simulink model "Template"  (R2018a)
settings: Solver=FixedStepDiscrete  StartTime=0.0  StopTime=0.001  RelTol=1e-3
values from neighbouring files (symbols this model uses):
  T = 1/Fs    (= 5e-05)    [SimVar.m]
undefined symbols (not defined in the file or in its folder): fdesignblkfcn, gcbh, get
libraries: dspsrcs4 x1, dspxfrm3 x1, dspobslib x1
settings Model: Creator=Daniel  LastModifiedBy=Daniel
settings SolverCC: AutoInsertRateTranBlk=on
settings DataIOCC: LimitDataPoints=on  SaveOutput=off  SignalLogging=off  SaveTime=off
settings OptimizationCC: LifeSpan=inf  SimCompilerOptimization=on
settings DebuggingCC: AlgebraicLoopMsg=error  SingleTaskRateTransMsg=error  AllowSymbolicDim=off  SFUnexpectedBacktrackingDiag=warning  SFNoUnconditionalDefaultTransitionDiag=warning  SFExecutionAtInitializationDiag=none
settings CodeAppCC: StateflowObjectComments=on
settings GRTTargetCC: TargetLangStandard=C89/C90 (ANSI)  GeneratePreprocessorConditionals=Disable all
settings ConfigComp: CovMetricSettings=dw  CovHtmlReporting=on  CovSaveCumulativeToWorkspaceVar=on  CovSaveSingleToWorkspaceVar=on  CovExternalEMLEnable=off  CovSFcnEnable=off

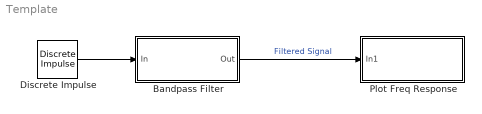
== system Template ==
  Bandpass Filter : Subsystem  DialogController=fdesignblkfcn  InitFcn=fdesignblkfcn(gcbh, {'InitFcn'});  mask(Bandpass Filter){}
      mask help: Design a bandpass filter
      settings: CopyFcn=fdesignblkfcn(gcbh, {'CopyFcn'});
      mask Help: helpview(mapfilelocation('dsp'), 'dspbandpassfilter');
      mask Display: disp('Bandpass');
  Discrete Impulse : dspsrcs4/Discrete  Impulse  Delay=0  SampleTime=T  FrameSample=128  OutputFrames=off  dataType=double  isSigned=on  wordLen=16  udDataType=sfix(16)  fracBitsMode=Best precision  numFracBits=15  OutDataTypeStr=double  LastOutDataTypeStr=double
  Plot Freq Response : Subsystem
  wires:
  Discrete Impulse/1 -> Bandpass Filter/1(In)
  Bandpass Filter/1(Out) -> Plot Freq Response/1(In1)  "Filtered Signal"

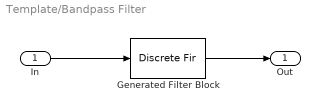
== system Template/Bandpass Filter ==
  In : Inport
  Generated Filter Block : DiscreteFir  Tag=BlockMethodSubSystem  Coefficients=[-0.0143829707087432795 -0.0290029983982484744 0.00784048811812495389 0.0308165601876585482 0.00100231088912336496 0.0087190389177637332 0.0151927377592376723 -0.00168387668084986558 0.0111183190197781962 0.00421002856557019852 0.000673765264122200562 0.00910146591908392137 -0.00227014796668174043 0.00546863785810260041 0.00231714434328688865 -0.00136078413445314315 0.00603880317721489351 -0.00343031068051817024 0.00347055870875673288 0.000464183487342060218 -0.00250956115928813303 0.00433762157606339387 -0.00498706380103555377 0.00246050102483365242 -0.00143811368573451407 -0.00366854398739842411 0.00299692463358692748 -0.00698080238922849181 0.0016607418180266374 -0.00363600133190109583 -0.00501339083555271074 0.00160027598954386673 -0.0094321788660009908 0.000886295582407861356 -0.00628897746187223605 -0.0065194850954027302 5.11766740212844773e-05 -0.0123554859169431042 0.000164116634503716995 -0.00940416859225592754 -0.00812346347120297338 -0.00168137988191204078 -0.015663036767903888 -0.000418207004173260346 -0.0130701898209931843 -0.00959179797111331389 -0.00355572086220254336 -0.0193608783369033331 -0.000521084234226450844 -0.0173133999523348084 -0.0107007240278947594 -0.00537625194890753704 -0.0234065514815256781 0.00019715747804796357 -0.0222943554071380022 -0.0110533490108922772 -0.00712479962423895764 -0.0279997831851122939 0.00247814575333669875 -0.0286390340403170698 -0.0100330097329494102 -0.00860241371700308857 -0.0337042027750407563 0.00792224655421421529 -0.0380065734612550499 -0.00595127288610197355 -0.00974757221495216666 -0.042872984118998099 0.0219305315464521679 -0.0575862054909740129 0.00748817667562471159 -0.010468068896780874 -0.0700145229057000801 0.0849475936329411874 -0.16679316932022728 0.163330198222631923 0.78931487915433507 0.163330198222631923 -0.16679316932022728 0.0849475936329411874 -0.0700145229057000801 -0.010468068896780874 0.00748817667562471159 -0.0575862054909740129 0.0219305315464521679 -0.042872984118998099 -0.00974757221495216666 -0.00595127288610197355 -0.0380065734612550499 0.00792224655421421529 -0.0337042027750407563 -0.00860241371700308857 -0.0100330097329494102 -0.0286390340403170698 0.00247814575333669875 -0.0279997831851122939 -0.00712479962423895764 -0.0110533490108922772 -0.0222943554071380022 0.00019715747804796357 -0.0234065514815256781 -0.00537625194890753704 -0.0107007240278947594 -0.0173133999523348084 -0.000521084234226450844 -0.0193608783369033331 -0.00355572086220254336 -0.00959179797111331389 -0.0130701898209931843 -0.000418207004173260346 -0.015663036767903888 -0.00168137988191204078 -0.00812346347120297338 -0.00940416859225592754 0.000164116634503716995 -0.0123554859169431042 5.11766740212844773e-05 -0.0065194850954027302 -0.00628897746187223605 0.000886295582407861356 -0.0094321788660009908 0.00160027598954386673 -0.00501339083555271074 -0.00363600133190109583 0.0016607418180266374 -0.00698080238922849181 0.00299692463358692748 -0.00366854398739842411 -0.00143811368573451407 0.00246050102483365242 -0.00498706380103555377 0.00433762157606339387 -0.00250956115928813303 0.000464183487342060218 0.00347055870875673288 -0.00343031068051817024 0.00603880317721489351 -0.00136078413445314315 0.00231714434328688865 0.00546863785810260041 -0.00227014796668174043 0.00910146591908392137 0.000673765264122200562 0.00421002856557019852 0.0111183190197781962 -0.00168387668084986558 0.0151927377592376723 0.0087190389177637332 0.00100231088912336496 0.0308165601876585482 0.00784048811812495389 -0.0290029983982484744 -0.0143829707087432795]  InputProcessing=Columns as channels (frame based)
  Out : Outport
  wires:
  In/1 -> Generated Filter Block/1
  Generated Filter Block/1 -> Out/1

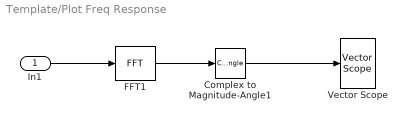
== system Template/Plot Freq Response ==
  In1 : Inport
  Complex to Magnitude-Angle1 : ComplexToMagnitudeAngle  Output=Magnitude
  FFT1 : dspxfrm3/FFT  FFTImplementation=Auto  CompMethod=Table lookup  TableOpt=NEW  TableOptActive=Speed  BitRevOrder=off  Normalize=off  InheritFFTLength=on  FFTLength=64  WrapInput=on  roundingMode=Floor  overflowMode=off  firstCoeffDataTypeStr=Inherit: Same word length as input  firstCoeffLastDataTypeStr=Inherit: Same word length as input  outputMin=[]  outputMax=[]
  Vector Scope : dspobslib/Vector Scope  ScopeProperties=off  Domain=Frequency  HorizSpan=1  DisplayProperties=off  AxisGrid=on  Memory=off  FrameNumber=on  AxisLegend=off  AxisZoom=off  OpenScopeAtSimStart=on  OpenScopeImmediately=off  FigPos=get(0,'defaultfigureposition')  AxisProperties=on  XUnits=Hertz  XRange=[0...Fs/2]  InheritXIncr=on  XIncr=1  XLabel=Samples  XLimit=Auto  XMin=0  XMax=1  XStart=0  YUnits=dB  YLabel=|Magnitude (dB)|  LineProperties=off  XAxisParamsVer=6.9
      settings: SourceProductName=DSP System Toolbox  SourceProductBaseCode=DS  YMin=0.0723692553519949  YMax=69.3188381671759
  wires:
  In1/1 -> FFT1/1
  FFT1/1 -> Complex to Magnitude-Angle1/1
  Complex to Magnitude-Angle1/1 -> Vector Scope/1
